simulink model "IMC_withoutboost"  (R2021b)
settings: Solver=VariableStepAuto  StartTime=0.0  StopTime=100  RelTol=1e-3
settings Model: Creator=ismt  LastModifiedBy=ismt

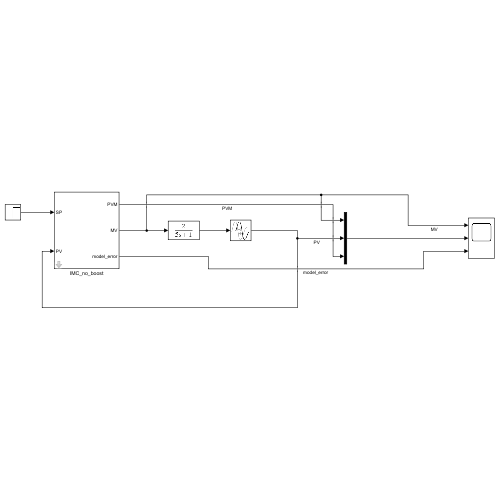
[thumbnail: Simulink's stored preview of the top-level diagram]
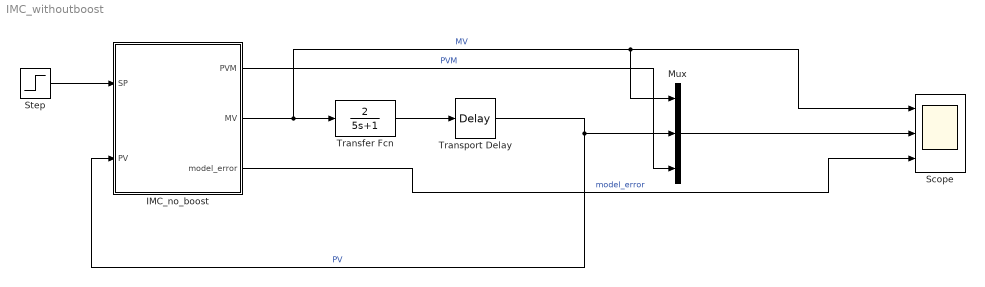
== system IMC_withoutboost ==
  IMC_no_boost : Subsystem  mask{Kp_hat=2, tau_hat=1, delay_hat=4}
  Mux : Mux  Inputs=3
  Scope : Scope  NumInputPorts=3
  Step : Step  After=10  SampleTime=0
  Transfer Fcn : TransferFcn  Numerator=[2]  Denominator=[5 1]
  Transport Delay : TransportDelay  DelayTime=2.5
  wires:
  IMC_no_boost/2(MV) -> Scope/1, Mux/1, Transfer Fcn/1  "MV"
  Transfer Fcn/1 -> Transport Delay/1
  Transport Delay/1 -> Mux/2, IMC_no_boost/2(PV)  "PV"
  IMC_no_boost/1(PVM) -> Mux/3  "PVM"
  Mux/1 -> Scope/2
  IMC_no_boost/3(model_error) -> Scope/3  "model_error"
  Step/1 -> IMC_no_boost/1(SP)

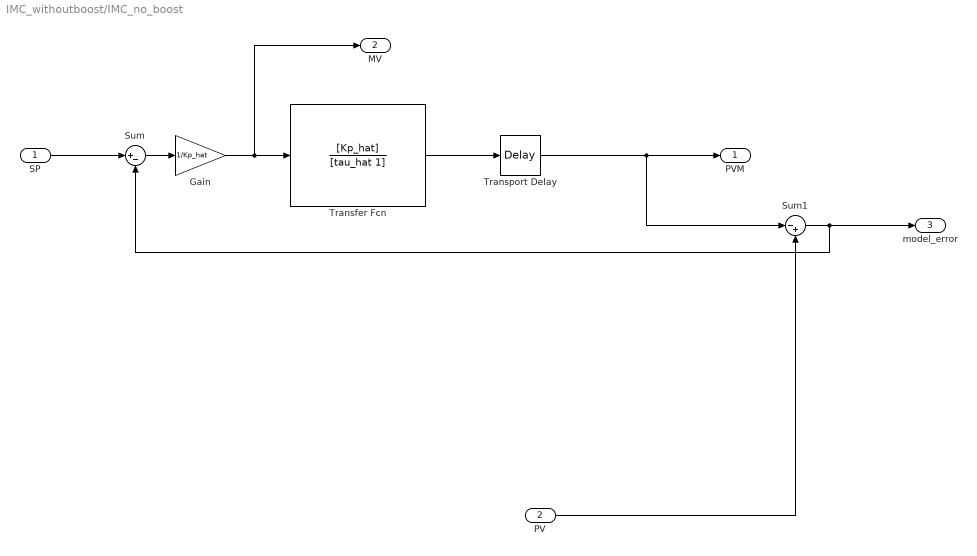
== system IMC_withoutboost/IMC_no_boost ==
  SP : Inport
  PV : Inport  Port=2
  Gain : Gain  Gain=1/Kp_hat
  Sum : Sum  Inputs=|+-
  Sum1 : Sum  Inputs=|-+
  Transfer Fcn : TransferFcn  Numerator=[Kp_hat]  Denominator=[tau_hat 1]
  Transport Delay : TransportDelay  DelayTime=delay_hat
  PVM : Outport
  MV : Outport  Port=2
  model_error : Outport  Port=3
  wires:
  Sum1/1 -> model_error/1, Sum/2
  Sum/1 -> Gain/1
  Gain/1 -> MV/1, Transfer Fcn/1
  Transfer Fcn/1 -> Transport Delay/1
  Transport Delay/1 -> PVM/1, Sum1/1
  SP/1 -> Sum/1
  PV/1 -> Sum1/2
